simulink model "Indirect_MRAC"  (R2014a)
settings: Solver=ode23t  StartTime=0.0  StopTime=100  RelTol=1e-3
settings Model: Creator=saura_000  LastModifiedBy=saura_000

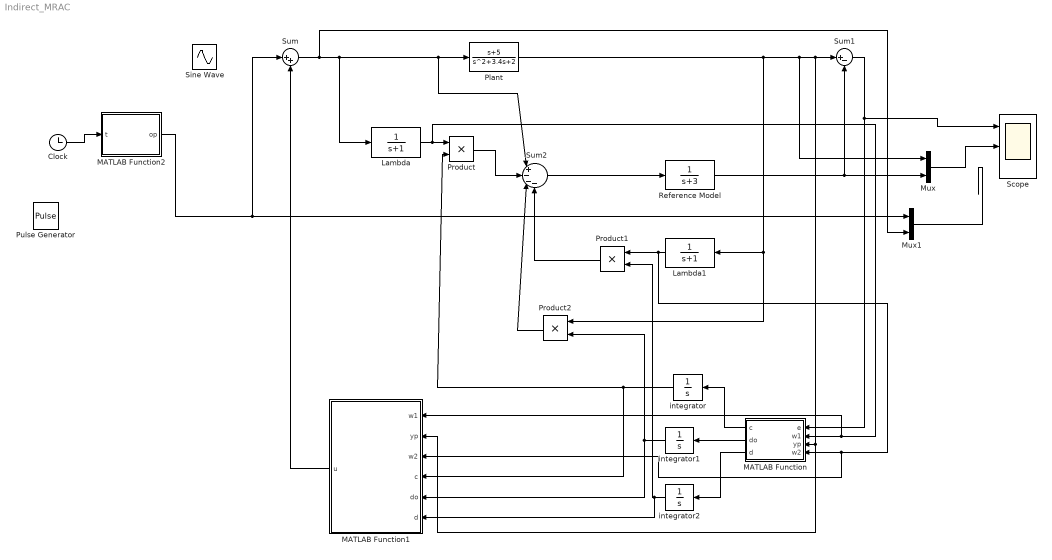
== system Indirect_MRAC ==
  Clock : Clock
  Lambda : TransferFcn  Denominator=[1 1]
  Lambda1 : TransferFcn  Denominator=[1 1]
  MATLAB Function : MATLAB Function  TreatAsAtomicUnit=on
  MATLAB Function1 : MATLAB Function  TreatAsAtomicUnit=on
  MATLAB Function2 : MATLAB Function  TreatAsAtomicUnit=on
  Mux : Mux  Inputs=2
  Mux1 : Mux  Inputs=2
  Plant : TransferFcn  Numerator=[1 5]  Denominator=[1 3.4 2]
  Product : Product
  Product1 : Product
  Product2 : Product
  Pulse Generator : DiscretePulseGenerator  PulseType=Time based  Amplitude=5  Period=0.2  PulseWidth=50
  Reference Model : TransferFcn  Denominator=[1 3]
  Scope : Scope  NumInputPorts=3
      settings: YMin=-5~-5~-5  YMax=5~5~5
  Sine Wave : Sin  Frequency=0.1*pi  SampleTime=0
  Sum : Sum  Inputs=|++
  Sum1 : Sum  Inputs=|+-
  Sum2 : Sum  Inputs=|+---
  integrator : TransferFcn  Denominator=[1 0]
  integrator1 : TransferFcn  Denominator=[1 0]
  integrator2 : TransferFcn  Denominator=[1 0]
  wires:
  Sum/1 -> Mux1/2, Lambda/1, Sum2/1, Plant/1
  Plant/1 -> Product2/1, Lambda1/1, Mux/1, MATLAB Function1/2(yp), MATLAB Function/3(yp), Sum1/1
  Lambda/1 -> MATLAB Function1/1(w1), MATLAB Function/2(w1), Product/1
  Product/1 -> Sum2/2
  Sum2/1 -> Reference Model/1
  Reference Model/1 -> Sum1/2, Mux/2
  Lambda1/1 -> MATLAB Function1/3(w2), MATLAB Function/4(w2), Product1/1
  Product1/1 -> Sum2/4
  Product2/1 -> Sum2/3
  Sum1/1 -> Scope/1, MATLAB Function/1(e)
  MATLAB Function/1(c) -> integrator/1
  MATLAB Function/2(do) -> integrator1/1
  MATLAB Function/3(d) -> integrator2/1
  integrator/1 -> MATLAB Function1/4(c), Product/2
  integrator1/1 -> Product2/2, MATLAB Function1/5(do)
  integrator2/1 -> MATLAB Function1/6(d), Product1/2
  MATLAB Function1/1(u) -> Sum/2
  MATLAB Function2/1(op) -> Sum/1, Mux1/1
  Mux/1 -> Scope/2
  Mux1/1 -> ?
  Clock/1 -> MATLAB Function2/1(t)

== matlab function Indirect_MRAC/MATLAB Function1 ==
  data: u output; w1 input; yp input; w2 input; c input; do input; d input
function u  = fcn(w1,yp,w2,c,do,d)
%#codegen
a = [c do d];
b = [w1 yp w2]';
u = a*b;

== matlab function Indirect_MRAC/MATLAB Function ==
  data: e input; c output; w1 input; yp input; w2 input; do output; d output
function [c,do,d] = fcn(e,w1,yp,w2)
c = -(e*w1);
do = -(e*yp);
d = -(e*w2);

== matlab function Indirect_MRAC/MATLAB Function2 ==
  data: t input; op output
function op  = fcn(t)
op = 5*cos(2*pi*t) + 10*cos(10*pi*t);
